simulink model "Full_avg_converter"  (R2023b)
settings: Solver=VariableStepAuto  StartTime=0.0  StopTime=sim_time  RelTol=1e-3
undefined symbols (not defined in the file or in its folder): Bat, boost, ccm_mpp_reg_param, ccm_reg_param, dcm_mpp_reg_param, dcm_reg_param, m0_ccm, mppt_my3, pv_data, pv_eq, Ramp, sim_op, Tmfc, Uoc_max, Uref
libraries: spsBistableLib x3, slpidlib x3, simulink x1, spspowerguiLib x1
settings Model: Creator=teo  LastModifiedBy=teo

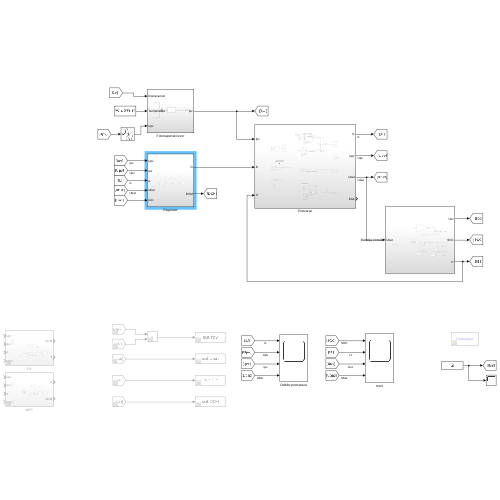
[thumbnail: Simulink's stored preview of the top-level diagram]
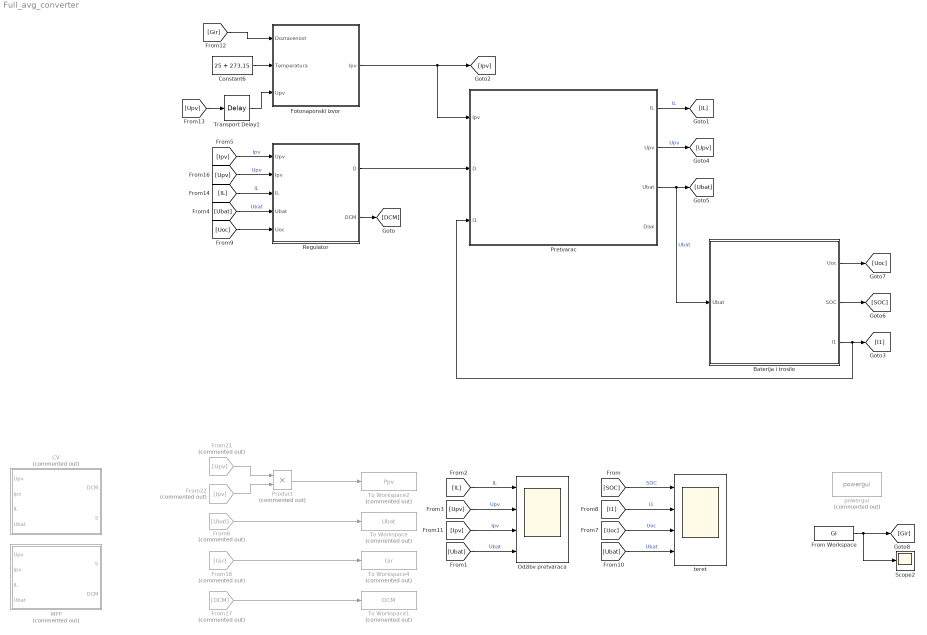
== system Full_avg_converter ==
  Baterija i trosilo : Subsystem
  CV : Subsystem  Commented=on
  Constant6 : Constant  Value=25 + 273.15
  Fotonaponski izvor : Subsystem
  From Workspace : FromWorkspace  VariableName=GI
  From17 : From  Commented=on  GotoTag=DCM
  From18 : From  Commented=on  GotoTag=Gir
  From21 : From  Commented=on  GotoTag=Upv
  From22 : From  Commented=on  GotoTag=Ipv
  From6 : From  Commented=on  GotoTag=Ubat
  MPP : Subsystem  Commented=on
  Odzibv pretvaraca : Scope  NumInputPorts=4
  Pretvarac : Subsystem
  Product : Product  Commented=on
  Regulator : Subsystem
  Scope2 : Scope
  To Workspace : ToWorkspace  Commented=on  VariableName=Ubat  SaveFormat=Timeseries  SampleTime=-1
  To Workspace1 : ToWorkspace  Commented=on  VariableName=DCM  SaveFormat=Timeseries  SampleTime=-1
  To Workspace2 : ToWorkspace  Commented=on  VariableName=Ppv  SaveFormat=Timeseries  SampleTime=-1
  To Workspace4 : ToWorkspace  Commented=on  VariableName=Gir  SaveFormat=Timeseries  SampleTime=-1
  Transport Delay1 : TransportDelay  DelayTime=0.0001  BufferSize=4024
  powergui : spspowerguiLib/powergui  Priority=1  Commented=on  SimulationMode=Continuous  SampleTime=50e-6  frequency=60  Iterations=50  frequencyindice=0  Pbase=100e6  ErrMax=1e-4  UnitsV=kV  UnitsW=MW  buscounter=0  FunctionMessages=off  echomessages=off  EnableUseOfTLC=off  CurrentSourceSwitches=off  DisableSnubberDevices=off  DisableRonSwitches=off  DisableVfSwitches=off  DisplayEquations=off  AutomaticDiscreteSolvers=off  SolverType=Tustin/Backward Euler (TBE)  Interpol=off  ExternalGateDelay=off  methode=off  Ts=100  x0status=blocks  SPID=on  SwTol=0  HookPort=off  NonlinearTolerance=1e-4  nMaxIteration=100  ContinueOnMaxIteration=off  RestoreLinks=warning  ResistiveCurrentMeasurement=off  Frange=[0:2:500]  Ylog=off  Xlog=on  ShowGrid=off  save=off  variable=ZData  structure=0  ZoomFFT=off  StartTime=0.0  cycles=1  DisplayStyle=1  fundamental=60  FreqAxis=off  MaxFrequency=1000  frequencyindicesteady=1  RmsSteady=1  display=off
  teret : Scope  NumInputPorts=4
  wires:
  Product/1 -> To Workspace2/1
  [I1] -> teret/2  "I1"
  Transport Delay1/1 -> Fotonaponski izvor/3(Upv)
  [Ubat] -> Odzibv pretvaraca/4  "Ubat"
  Constant6/1 -> Fotonaponski izvor/2(Temperatura)
  [Upv] -> Odzibv pretvaraca/2  "Upv"
  From Workspace/1 -> Scope2/1, [Gir]
  [Upv] -> Transport Delay1/1
  [Ipv] -> Odzibv pretvaraca/3  "Ipv"
  [Ubat] -> teret/4  "Ubat"
  From18/1 -> To Workspace4/1
  [IL] -> Odzibv pretvaraca/1  "IL"
  From6/1 -> To Workspace/1
  From17/1 -> To Workspace1/1
  From21/1 -> Product/1
  From22/1 -> Product/2
  Regulator/1(D) -> Pretvarac/2(D)
  Regulator/2(DCM) -> [DCM]
  [IL] -> Regulator/3(IL)  "IL"
  [Ubat] -> Regulator/4(Ubat)  "Ubat"
  [Upv] -> Regulator/2(Ipv)  "Upv"
  [Ipv] -> Regulator/1(Upv)  "Ipv"
  Pretvarac/1(IL) -> [IL]  "IL"
  Pretvarac/2(Upv) -> [Upv]  "Upv"
  Pretvarac/3(Ubat) -> Baterija i trosilo/1(Ubat), [Ubat]  "Ubat"
  Baterija i trosilo/3(I1) -> [I1], Pretvarac/3(I1)
  Baterija i trosilo/2(SOC) -> [SOC]
  Fotonaponski izvor/1(Ipv) -> [Ipv], Pretvarac/1(Ipv)
  Baterija i trosilo/1(Uoc) -> [Uoc]
  [Uoc] -> Regulator/5(Uoc)
  [SOC] -> teret/1  "SOC"
  [Uoc] -> teret/3  "Uoc"
  [Gir] -> Fotonaponski izvor/1(Dozracenost)

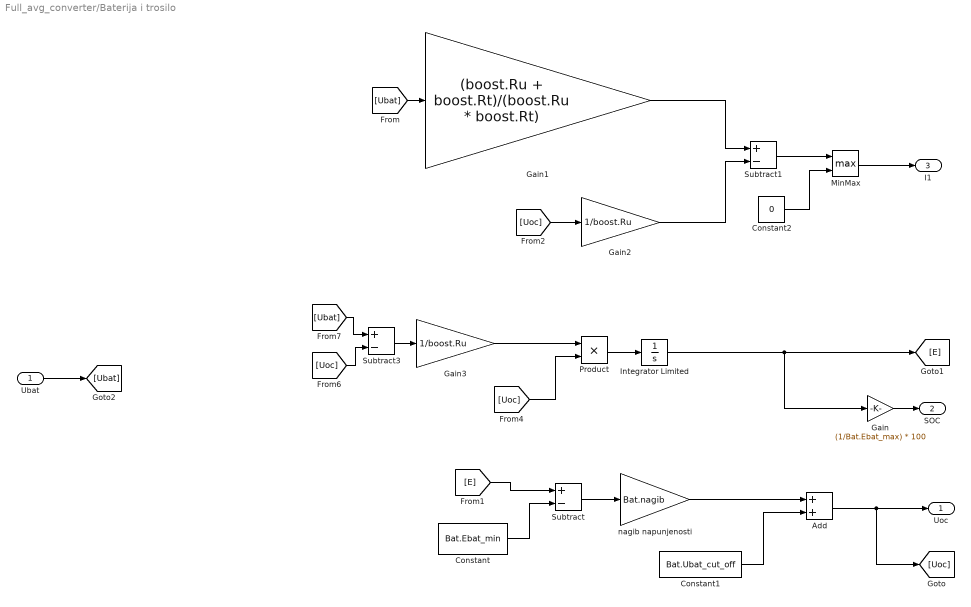
== system Full_avg_converter/Baterija i trosilo ==
  Ubat : Inport
  Add : Sum
  Constant : Constant  Value=Bat.Ebat_min
  Constant1 : Constant  Value=Bat.Ubat_cut_off
  Constant2 : Constant  Value=0
  Gain : Gain  Gain=(1/Bat.Ebat_max) * 100
  Gain1 : Gain  Gain=(boost.Ru + boost.Rt)/(boost.Ru * boost.Rt)
  Gain2 : Gain  Gain=1/boost.Ru
  Gain3 : Gain  Gain=1/boost.Ru
  Integrator Limited : Integrator  InitialCondition=sim_op.E0  LimitOutput=on  UpperSaturationLimit=Bat.Ebat_max  LowerSaturationLimit=Bat.Ebat_min
  MinMax : MinMax  Function=max  Inputs=2
  Product : Product
  Subtract : Sum  Inputs=+-
  Subtract1 : Sum  Inputs=+-
  Subtract3 : Sum  Inputs=+-
  nagib napunjenosti : Gain  Gain=Bat.nagib
  Uoc : Outport
  SOC : Outport  Port=2
  I1 : Outport  Port=3
  wires:
  Subtract/1 -> nagib napunjenosti/1
  Constant/1 -> Subtract/2
  nagib napunjenosti/1 -> Add/1
  Constant1/1 -> Add/2
  Integrator Limited/1 -> Gain/1, [E]
  [Uoc] -> Product/2
  Product/1 -> Integrator Limited/1
  [E] -> Subtract/1
  Gain/1 -> SOC/1
  Add/1 -> Uoc/1, [Uoc]
  Ubat/1 -> [Ubat]
  [Ubat] -> Gain1/1
  Gain1/1 -> Subtract1/1
  [Uoc] -> Gain2/1
  Gain2/1 -> Subtract1/2
  MinMax/1 -> I1/1
  Subtract1/1 -> MinMax/1
  Constant2/1 -> MinMax/2
  Subtract3/1 -> Gain3/1
  Gain3/1 -> Product/1
  [Ubat] -> Subtract3/1
  [Uoc] -> Subtract3/2

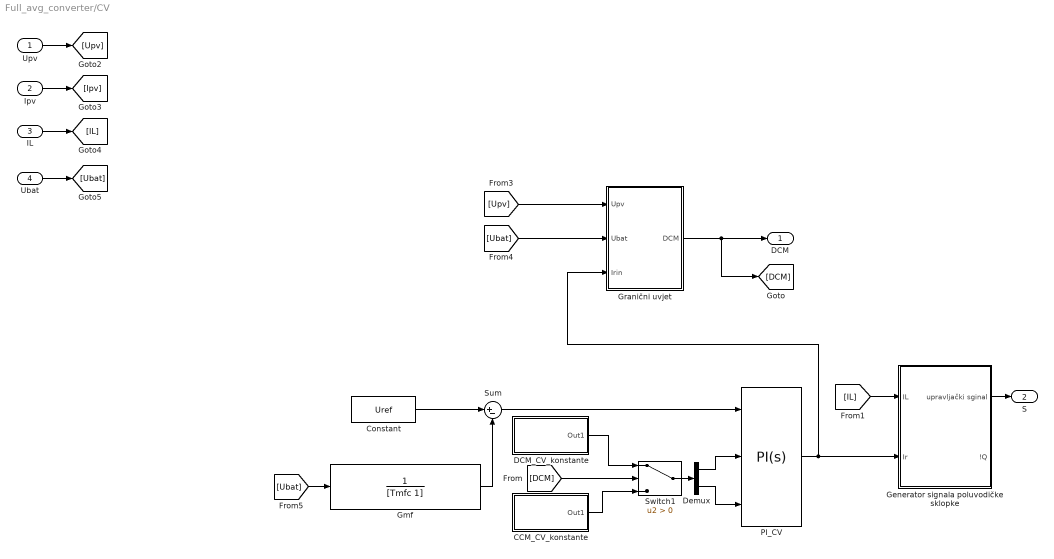
== system Full_avg_converter/CV ==
  Upv : Inport
  Ipv : Inport  Port=2
  IL : Inport  Port=3
  Ubat : Inport  Port=4
  CCM_CV_konstante : Subsystem
  Constant : Constant  Value=Uref
  DCM_CV_konstante : Subsystem
  Demux : Demux  Outputs=2
  Generator signala poluvodičke sklopke : Subsystem
  Gmf : TransferFcn  Numerator=1  Denominator=[Tmfc 1]
  Granični uvjet : Subsystem
  PI_CV : slpidlib/PID Controller  Controller=PI  Form=Parallel  TimeDomain=Continuous-time  UseExternalTs=off  SampleTime=-1  IntegratorMethod=Forward Euler  FilterMethod=Forward Euler  ControllerParametersSource=external  P=ccm_mpp_reg_param.KR  I=ccm_mpp_reg_param.KR/ccm_mpp_reg_param.Ti  UseKiTs=off  D=0  N=100  UseFilter=on  TunerSelectOption=Transfer Function Based (PID Tuner App)  InitialConditionSource=internal  InitialConditionForIntegrator=0  InitialConditionForFilter=0  DifferentiatorICPrevScaledInput=0  ExternalReset=none  TrackingMode=off  Kt=1  LimitOutput=on  SatLimitsSource=internal  UpperSaturationLimit=2  LowerSaturationLimit=-2  LinearizeAsGain=off  AntiWindupMode=clamping  Kb=1  LimitIntegrator=off  UpperIntegratorSaturationLimit=inf  LowerIntegratorSaturationLimit=-inf  POutMin=[]  POutMax=[]  IOutMin=[]  IOutMax=[]  DOutMin=[]  DOutMax=[]  NOutMin=[]  NOutMax=[]  SumOutMin=[]  SumOutMax=[]  SaturationOutMin=[]  SaturationOutMax=[]  PParamMin=[]  PParamMax=[]  IParamMin=[]  IParamMax=[]  DParamMin=[]  DParamMax=[]  NParamMin=[]  NParamMax=[]  KbParamMin=[]  KbParamMax=[]  KtParamMin=[]  KtParamMax=[]  KbOutMin=[]  KbOutMax=[]  KtOutMin=[]  KtOutMax=[]  IntegratorOutMin=[]  IntegratorOutMax=[]  FilterOutMin=[]  FilterOutMax=[]  SumI1OutMin=[]  SumI1OutMax=[]  SumI2OutMin=[]  SumI2OutMax=[]  SumI3OutMin=[]  SumI3OutMax=[]  SumI4OutMin=[]  SumI4OutMax=[]  SumDOutMin=[]  SumDOutMax=[]  DifferentiatorOutMin=[]  DifferentiatorOutMax=[]  FilterDiffOutCoefMin=[]  FilterDiffOutCoefMax=[]  ReciprocalOutMin=[]  ReciprocalOutMax=[]  SumDenOutMin=[]  SumDenOutMax=[]  SumNumOutMin=[]  SumNumOutMax=[]  DivideOutMin=[]  DivideOutMax=[]  UdiffTsProdOutMin=[]  UdiffTsProdOutMax=[]  NTsProdOutMin=[]  NTsProdOutMax=[]  UintegralTsProdOutMin=[]  UintegralTsProdOutMax=[]  UngainTsProdOutMin=[]  UngainTsProdOutMax=[]  ClampingZeroOutDataTypeStr=Inherit: Inherit via back propagation  ClampingZeroOutMin=[]  ClampingZeroOutMax=[]  FilterDenConstantOutDataTypeStr=Inherit: Inherit via back propagation  FilterDenConstantOutMin=[]  FilterDenConstantOutMax=[]  PCopyOutDataTypeStr=Inherit: Inherit via back propagation  PCopyOutMin=[]  PCopyOutMax=[]  NCopyOutDataTypeStr=Inherit: Inherit via back propagation  NCopyOutMin=[]  NCopyOutMax=[]  IntegratorContinuousStateAttributes=''  IntegratorStateMustResolveToSignalObject=off  IntegratorRTWStateStorageClass=Auto  FilterContinuousStateAttributes=''  FilterStateMustResolveToSignalObject=off  FilterRTWStateStorageClass=Auto  ParallelPVariant=ExternalParameters  IdealPVariant=Disabled  IVariant=ExternalParameters  DVariant=Disabled  IntegratorVariant=Continuous  SatVariant=Enabled  AWVariant=ContClampingParallel  PCopyVariant=Disabled  TRVariant=Disabled  FdbkBlocksVariant=Forward  IdealPFdbkVariant=Disabled  SatFdbkVariant=Disabled  DerivativeFilterVariant=Disabled  NVariant=Disabled  NCopyVariant=Disabled_SignalSpec  FilterICVariant=Disabled  IntegratorICVariant=InternalICs  ExternalResetVariant=Disabled  TRSumVariant=Passthrough  SumFdbkVariant=Disabled  SumVariant=Sum_PI  TsampFilterVariant=InternalTs  TsampNgainVariant=Passthrough  TsampIntegralVariant=Disabled_SignalSpec  ExternalSaturationOutDataTypeStr=Inherit: Same as second input
  Sum : Sum  Inputs=|+-
  Switch1 : Switch  Criteria=u2 > Threshold  SaturateOnIntegerOverflow=off  InputSameDT=off
  DCM : Outport
  S : Outport  Port=2
  wires:
  Switch1/1 -> Demux/1
  Demux/1 -> PI_CV/2
  Demux/2 -> PI_CV/3
  [DCM] -> Switch1/2
  DCM_CV_konstante/1(Out1) -> Switch1/1
  CCM_CV_konstante/1(Out1) -> Switch1/3
  Generator signala poluvodičke sklopke/1(upravljački sginal) -> S/1
  Upv/1 -> [Upv]
  Ipv/1 -> [Ipv]
  Ubat/1 -> [Ubat]
  IL/1 -> [IL]
  Granični uvjet/1(DCM) -> [DCM], DCM/1
  [Upv] -> Granični uvjet/1(Upv)
  [Ubat] -> Granični uvjet/2(Ubat)
  PI_CV/1 -> Generator signala poluvodičke sklopke/2(Ir), Granični uvjet/3(Irin)
  [IL] -> Generator signala poluvodičke sklopke/1(IL)
  [Ubat] -> Gmf/1
  Constant/1 -> Sum/1
  Gmf/1 -> Sum/2
  Sum/1 -> PI_CV/1

== system Full_avg_converter/Fotonaponski izvor ==
  Dozracenost : Inport
  Temperatura : Inport  Port=2
  Upv : Inport  Port=3
  Fotonaponsko polje : MATLABFcn  MATLABFcn=pv_eq(u(1), u(2), [], u(3), pv_data, 1, 1)  OutputDimensions=1
  Mux : Mux  Inputs=3
  Ipv : Outport
  wires:
  Fotonaponsko polje/1 -> Ipv/1  "Ipv"
  Mux/1 -> Fotonaponsko polje/1
  Dozracenost/1 -> Mux/1
  Temperatura/1 -> Mux/2
  Upv/1 -> Mux/3

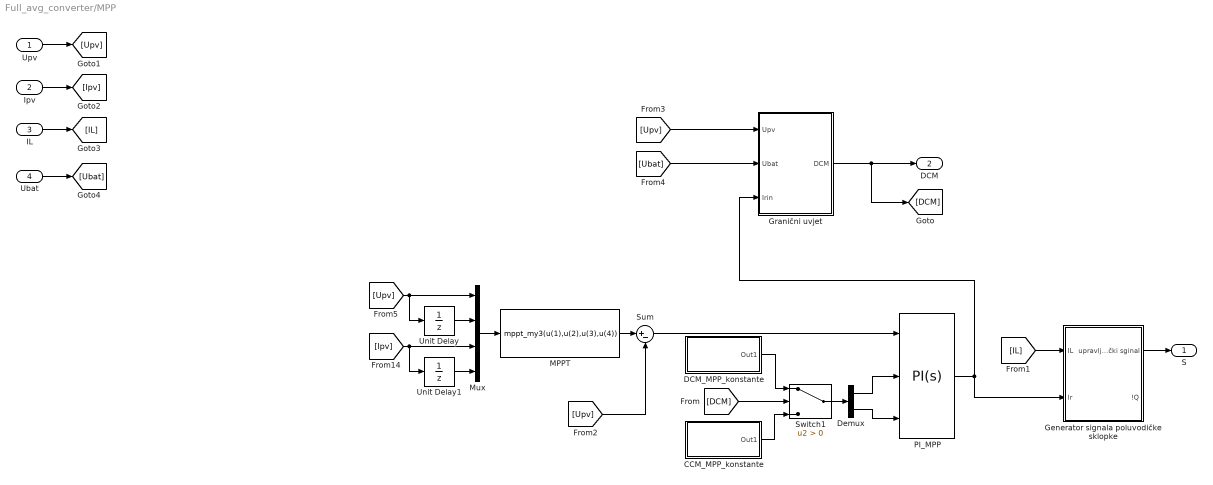
== system Full_avg_converter/MPP ==
  Upv : Inport
  Ipv : Inport  Port=2
  IL : Inport  Port=3
  Ubat : Inport  Port=4
  CCM_MPP_konstante : Subsystem
  DCM_MPP_konstante : Subsystem
  Demux : Demux  Outputs=2
  Generator signala poluvodičke sklopke : Subsystem
  Granični uvjet : Subsystem
  MPPT : MATLABFcn  MATLABFcn=mppt_my3(u(1),u(2),u(3),u(4))
  Mux : Mux
  PI_MPP : slpidlib/PID Controller  Controller=PI  Form=Parallel  TimeDomain=Continuous-time  UseExternalTs=off  SampleTime=-1  IntegratorMethod=Forward Euler  FilterMethod=Forward Euler  ControllerParametersSource=external  P=ccm_mpp_reg_param.KR  I=ccm_mpp_reg_param.KR/ccm_mpp_reg_param.Ti  UseKiTs=off  D=0  N=100  UseFilter=on  TunerSelectOption=Transfer Function Based (PID Tuner App)  InitialConditionSource=internal  InitialConditionForIntegrator=0  InitialConditionForFilter=0  DifferentiatorICPrevScaledInput=0  ExternalReset=none  TrackingMode=off  Kt=1  LimitOutput=on  SatLimitsSource=internal  UpperSaturationLimit=2  LowerSaturationLimit=-2  LinearizeAsGain=off  AntiWindupMode=clamping  Kb=1  LimitIntegrator=off  UpperIntegratorSaturationLimit=inf  LowerIntegratorSaturationLimit=-inf  POutMin=[]  POutMax=[]  IOutMin=[]  IOutMax=[]  DOutMin=[]  DOutMax=[]  NOutMin=[]  NOutMax=[]  SumOutMin=[]  SumOutMax=[]  SaturationOutMin=[]  SaturationOutMax=[]  PParamMin=[]  PParamMax=[]  IParamMin=[]  IParamMax=[]  DParamMin=[]  DParamMax=[]  NParamMin=[]  NParamMax=[]  KbParamMin=[]  KbParamMax=[]  KtParamMin=[]  KtParamMax=[]  KbOutMin=[]  KbOutMax=[]  KtOutMin=[]  KtOutMax=[]  IntegratorOutMin=[]  IntegratorOutMax=[]  FilterOutMin=[]  FilterOutMax=[]  SumI1OutMin=[]  SumI1OutMax=[]  SumI2OutMin=[]  SumI2OutMax=[]  SumI3OutMin=[]  SumI3OutMax=[]  SumI4OutMin=[]  SumI4OutMax=[]  SumDOutMin=[]  SumDOutMax=[]  DifferentiatorOutMin=[]  DifferentiatorOutMax=[]  FilterDiffOutCoefMin=[]  FilterDiffOutCoefMax=[]  ReciprocalOutMin=[]  ReciprocalOutMax=[]  SumDenOutMin=[]  SumDenOutMax=[]  SumNumOutMin=[]  SumNumOutMax=[]  DivideOutMin=[]  DivideOutMax=[]  UdiffTsProdOutMin=[]  UdiffTsProdOutMax=[]  NTsProdOutMin=[]  NTsProdOutMax=[]  UintegralTsProdOutMin=[]  UintegralTsProdOutMax=[]  UngainTsProdOutMin=[]  UngainTsProdOutMax=[]  ClampingZeroOutDataTypeStr=Inherit: Inherit via back propagation  ClampingZeroOutMin=[]  ClampingZeroOutMax=[]  FilterDenConstantOutDataTypeStr=Inherit: Inherit via back propagation  FilterDenConstantOutMin=[]  FilterDenConstantOutMax=[]  PCopyOutDataTypeStr=Inherit: Inherit via back propagation  PCopyOutMin=[]  PCopyOutMax=[]  NCopyOutDataTypeStr=Inherit: Inherit via back propagation  NCopyOutMin=[]  NCopyOutMax=[]  IntegratorContinuousStateAttributes=''  IntegratorStateMustResolveToSignalObject=off  IntegratorRTWStateStorageClass=Auto  FilterContinuousStateAttributes=''  FilterStateMustResolveToSignalObject=off  FilterRTWStateStorageClass=Auto  ParallelPVariant=ExternalParameters  IdealPVariant=Disabled  IVariant=ExternalParameters  DVariant=Disabled  IntegratorVariant=Continuous  SatVariant=Enabled  AWVariant=ContClampingParallel  PCopyVariant=Disabled  TRVariant=Disabled  FdbkBlocksVariant=Forward  IdealPFdbkVariant=Disabled  SatFdbkVariant=Disabled  DerivativeFilterVariant=Disabled  NVariant=Disabled  NCopyVariant=Disabled_SignalSpec  FilterICVariant=Disabled  IntegratorICVariant=InternalICs  ExternalResetVariant=Disabled  TRSumVariant=Passthrough  SumFdbkVariant=Disabled  SumVariant=Sum_PI  TsampFilterVariant=InternalTs  TsampNgainVariant=Passthrough  TsampIntegralVariant=Disabled_SignalSpec  ExternalSaturationOutDataTypeStr=Inherit: Same as second input
  Sum : Sum  Inputs=|+-
  Switch1 : Switch  Criteria=u2 > Threshold  SaturateOnIntegerOverflow=off  InputSameDT=off
  Unit Delay : UnitDelay  SampleTime=-1  HasFrameUpgradeWarning=on
  Unit Delay1 : UnitDelay  SampleTime=-1  HasFrameUpgradeWarning=on
  S : Outport
  DCM : Outport  Port=2
  wires:
  Switch1/1 -> Demux/1
  Demux/1 -> PI_MPP/2
  Demux/2 -> PI_MPP/3
  [DCM] -> Switch1/2
  DCM_MPP_konstante/1(Out1) -> Switch1/1
  CCM_MPP_konstante/1(Out1) -> Switch1/3
  PI_MPP/1 -> Granični uvjet/3(Irin), Generator signala poluvodičke sklopke/2(Ir)
  Generator signala poluvodičke sklopke/1(upravljački sginal) -> S/1
  Mux/1 -> MPPT/1
  Granični uvjet/1(DCM) -> [DCM], DCM/1
  MPPT/1 -> Sum/1
  [Upv] -> Sum/2
  Unit Delay/1 -> Mux/2
  Unit Delay1/1 -> Mux/4
  Sum/1 -> PI_MPP/1
  Upv/1 -> [Upv]
  Ipv/1 -> [Ipv]
  IL/1 -> [IL]
  Ubat/1 -> [Ubat]
  [IL] -> Generator signala poluvodičke sklopke/1(IL)
  [Upv] -> Granični uvjet/1(Upv)
  [Ubat] -> Granični uvjet/2(Ubat)
  [Upv] -> Unit Delay/1, Mux/1
  [Ipv] -> Unit Delay1/1, Mux/3

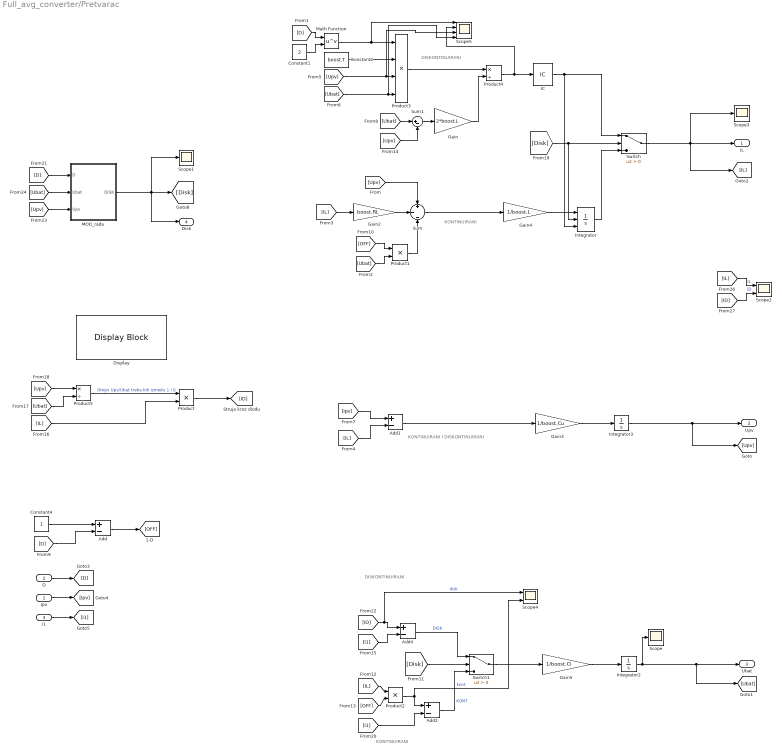
== system Full_avg_converter/Pretvarac ==
  note: DISKONTINUIRANI
  note: KONTINUIRANI
  note: KONTINUIRANI I DISKONTINUIRANI
  note: KONTINUIRANI
  note: DISKONTINUIRANI
  Ipv : Inport
  D : Inport  Port=2
  I1 : Inport  Port=3
  Add{,1..2,4} (4 alike) : Sum  Inputs=+-
  Constant1 : Constant  Value=2
  Constant2 : Constant  Value=boost.T
  Constant4 : Constant
  Display : DisplayBlock  LabelPosition=Bottom  Transparency=1
  Gain : Gain  Gain=2*boost.L
  Gain2 : Gain  Gain=boost.RL
  Gain3 : Gain  Gain=1/boost.Cu
  Gain4 : Gain  Gain=1/boost.L
  Gain5 : Gain  Gain=1/boost.Ci
  IC : InitialCondition  Value=0.1
  Integrator : Integrator  ExternalReset=falling  InitialConditionSource=external  LimitOutput=on  UpperSaturationLimit=150  LowerSaturationLimit=0
  Integrator2 : Integrator  InitialCondition=0.2  UpperSaturationLimit=Uoc_max + 10  LowerSaturationLimit=0
  Integrator3 : Integrator  InitialCondition=0.1  LimitOutput=on  UpperSaturationLimit=pv_data.Uoc  LowerSaturationLimit=0
  MOD_rada : Subsystem
  Math Function : Math  Operator=pow
  Product : Product
  Product1 : Product
  Product2 : Product
  Product3 : Product  Inputs=4
  Product4 : Product  Inputs=*/
  Product5 : Product  Inputs=*/
  Scope : Scope
  Scope1 : Scope
  Scope2 : Scope  NumInputPorts=2
  Scope3 : Scope
  Scope4 : Scope  NumInputPorts=2
  Scope5 : Scope  NumInputPorts=4
  Sum : Sum  Inputs=+|-|-
  Sum1 : Sum  Inputs=|+-
  Switch : Switch  Criteria=u2 > Threshold  SaturateOnIntegerOverflow=off  InputSameDT=off
  Switch1 : Switch  Criteria=u2 > Threshold  SaturateOnIntegerOverflow=off  InputSameDT=off
  IL : Outport
  Upv : Outport  Port=2
  Ubat : Outport  Port=3
  Disk : Outport  Port=4
  wires:
  I1/1 -> [I1]
  [Ipv] -> Add1/1
  D/1 -> [D]
  Ipv/1 -> [Ipv]
  [Upv] -> Sum/1
  [D] -> Add/2
  Constant4/1 -> Add/1
  Product1/1 -> Sum/3
  [OFF] -> Product1/1
  [Ubat] -> Product1/2
  [IL] -> Add1/2
  Sum/1 -> Gain4/1
  Add1/1 -> Gain3/1
  [D] -> Math Function/1
  Constant1/1 -> Math Function/2
  Math Function/1 -> Scope5/1, Product3/1
  Constant2/1 -> Product3/2
  [Upv] -> Scope5/3, Product3/3
  [Ubat] -> Scope5/4, Product3/4
  Product3/1 -> Product4/1
  [Ubat] -> Sum1/1
  [Upv] -> Sum1/2
  Sum1/1 -> Gain/1
  Gain3/1 -> Integrator3/1
  Gain/1 -> Product4/2
  Switch/1 -> Scope3/1, IL/1, [IL]
  Add/1 -> [OFF]
  Gain2/1 -> Sum/2
  [IL] -> Gain2/1
  Gain5/1 -> Integrator2/1
  [D] -> MOD_rada/1(D)
  [Upv] -> MOD_rada/3(Upv)
  [Ubat] -> MOD_rada/2(Ubat)
  Integrator3/1 -> [Upv], Upv/1
  Gain4/1 -> Integrator/1
  Integrator/1 -> Switch/3
  [Disk] -> Integrator/2, Switch/2
  [Upv] -> Product5/1
  [Ubat] -> Product5/2
  [IL] -> Product/2
  Product/1 -> [ID]
  Product5/1 -> Product/1  "Omjer Upv/Ubat treba biti izmedu 1 i 0"
  [ID] -> Scope4/1, Add4/1  "disk"
  [I1] -> Add4/2
  [IL] -> Scope2/1  "IL"
  [ID] -> Scope2/2  "ID"
  IC/1 -> Integrator/3, Switch/1
  Switch1/1 -> Gain5/1
  Add4/1 -> Switch1/1  "DISK"
  [Disk] -> Switch1/2
  [IL] -> Product2/1
  [OFF] -> Product2/2
  Product2/1 -> Add2/1, Scope4/2  "kont"
  [I1] -> Add2/2
  Add2/1 -> Switch1/3  "KONT"
  MOD_rada/1(DISK) -> Disk/1, Scope1/1, [Disk]
  Integrator2/1 -> [Ubat], Ubat/1, Scope/1
  Product4/1 -> Scope5/2, IC/1

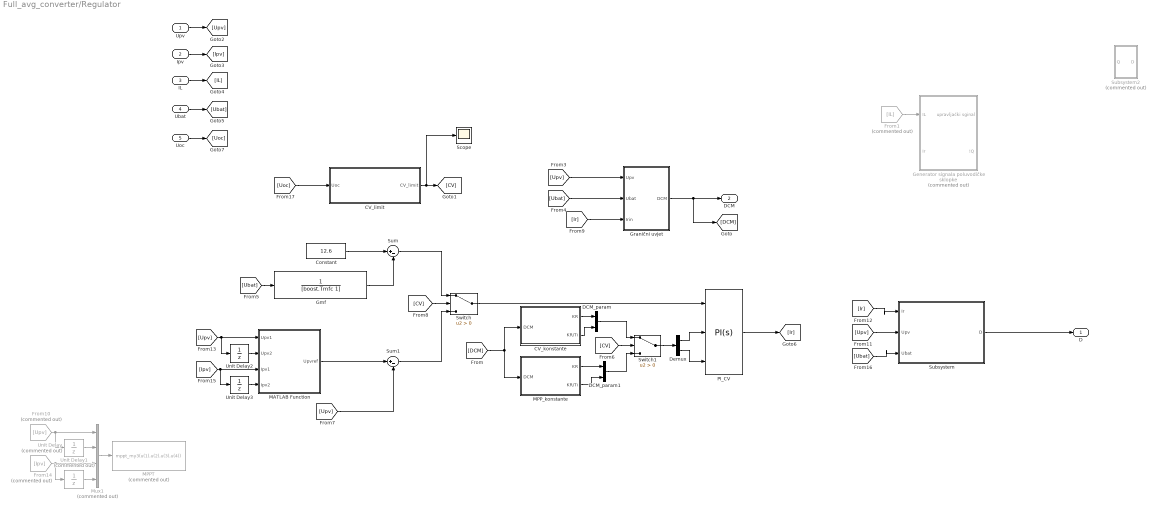
== system Full_avg_converter/Regulator ==
  Upv : Inport
  Ipv : Inport  Port=2
  IL : Inport  Port=3
  Ubat : Inport  Port=4
  Uoc : Inport  Port=5
  CV_konstante : Subsystem
  CV_limit : Subsystem
  Constant : Constant  Value=12.6
  DCM_param : Mux  Inputs=2
  DCM_param1 : Mux  Inputs=2
  Demux : Demux  Outputs=2
  From1 : From  Commented=on  GotoTag=IL
  From10 : From  Commented=on  GotoTag=Upv
  From14 : From  Commented=on  GotoTag=Ipv
  Generator signala poluvodičke sklopke : Subsystem  Commented=on
  Gmf : TransferFcn  Numerator=1  Denominator=[boost.Tmfc 1]
  Granični uvjet : Subsystem
  MATLAB Function : MATLAB Function  TreatAsAtomicUnit=on
  MPPT : MATLABFcn  Commented=on  MATLABFcn=mppt_my3(u(1),u(2),u(3),u(4))
  MPP_konstante : Subsystem
  Mux1 : Mux  Commented=on
  PI_CV : slpidlib/PID Controller  Controller=PI  Form=Parallel  TimeDomain=Continuous-time  UseExternalTs=off  SampleTime=-1  IntegratorMethod=Forward Euler  FilterMethod=Forward Euler  ControllerParametersSource=external  P=ccm_mpp_reg_param.KR  I=ccm_mpp_reg_param.KR/ccm_mpp_reg_param.Ti  UseKiTs=off  D=0  N=100  UseFilter=on  TunerSelectOption=Transfer Function Based (PID Tuner App)  InitialConditionSource=internal  InitialConditionForIntegrator=0  InitialConditionForFilter=0  DifferentiatorICPrevScaledInput=0  ExternalReset=none  TrackingMode=off  Kt=1  LimitOutput=on  SatLimitsSource=internal  UpperSaturationLimit=2  LowerSaturationLimit=-2  LinearizeAsGain=off  AntiWindupMode=clamping  Kb=1  LimitIntegrator=off  UpperIntegratorSaturationLimit=inf  LowerIntegratorSaturationLimit=-inf  POutMin=[]  POutMax=[]  IOutMin=[]  IOutMax=[]  DOutMin=[]  DOutMax=[]  NOutMin=[]  NOutMax=[]  SumOutMin=[]  SumOutMax=[]  SaturationOutMin=[]  SaturationOutMax=[]  PParamMin=[]  PParamMax=[]  IParamMin=[]  IParamMax=[]  DParamMin=[]  DParamMax=[]  NParamMin=[]  NParamMax=[]  KbParamMin=[]  KbParamMax=[]  KtParamMin=[]  KtParamMax=[]  KbOutMin=[]  KbOutMax=[]  KtOutMin=[]  KtOutMax=[]  IntegratorOutMin=[]  IntegratorOutMax=[]  FilterOutMin=[]  FilterOutMax=[]  SumI1OutMin=[]  SumI1OutMax=[]  SumI2OutMin=[]  SumI2OutMax=[]  SumI3OutMin=[]  SumI3OutMax=[]  SumI4OutMin=[]  SumI4OutMax=[]  SumDOutMin=[]  SumDOutMax=[]  DifferentiatorOutMin=[]  DifferentiatorOutMax=[]  FilterDiffOutCoefMin=[]  FilterDiffOutCoefMax=[]  ReciprocalOutMin=[]  ReciprocalOutMax=[]  SumDenOutMin=[]  SumDenOutMax=[]  SumNumOutMin=[]  SumNumOutMax=[]  DivideOutMin=[]  DivideOutMax=[]  UdiffTsProdOutMin=[]  UdiffTsProdOutMax=[]  NTsProdOutMin=[]  NTsProdOutMax=[]  UintegralTsProdOutMin=[]  UintegralTsProdOutMax=[]  UngainTsProdOutMin=[]  UngainTsProdOutMax=[]  ClampingZeroOutDataTypeStr=Inherit: Inherit via back propagation  ClampingZeroOutMin=[]  ClampingZeroOutMax=[]  FilterDenConstantOutDataTypeStr=Inherit: Inherit via back propagation  FilterDenConstantOutMin=[]  FilterDenConstantOutMax=[]  PCopyOutDataTypeStr=Inherit: Inherit via back propagation  PCopyOutMin=[]  PCopyOutMax=[]  NCopyOutDataTypeStr=Inherit: Inherit via back propagation  NCopyOutMin=[]  NCopyOutMax=[]  IntegratorContinuousStateAttributes=''  IntegratorStateMustResolveToSignalObject=off  IntegratorRTWStateStorageClass=Auto  FilterContinuousStateAttributes=''  FilterStateMustResolveToSignalObject=off  FilterRTWStateStorageClass=Auto  ParallelPVariant=ExternalParameters  IdealPVariant=Disabled  IVariant=ExternalParameters  DVariant=Disabled  IntegratorVariant=Continuous  SatVariant=Enabled  AWVariant=ContClampingParallel  PCopyVariant=Disabled  TRVariant=Disabled  FdbkBlocksVariant=Forward  IdealPFdbkVariant=Disabled  SatFdbkVariant=Disabled  DerivativeFilterVariant=Disabled  NVariant=Disabled  NCopyVariant=Disabled_SignalSpec  FilterICVariant=Disabled  IntegratorICVariant=InternalICs  ExternalResetVariant=Disabled  TRSumVariant=Passthrough  SumFdbkVariant=Disabled  SumVariant=Sum_PI  TsampFilterVariant=InternalTs  TsampNgainVariant=Passthrough  TsampIntegralVariant=Disabled_SignalSpec  ExternalSaturationOutDataTypeStr=Inherit: Same as second input
  Scope : Scope
  Subsystem : Subsystem
  Subsystem2 : Subsystem  Commented=on
  Sum : Sum  Inputs=|+-
  Sum1 : Sum  Inputs=|+-
  Switch : Switch  Criteria=u2 > Threshold  SaturateOnIntegerOverflow=off  InputSameDT=off
  Switch1 : Switch  Criteria=u2 > Threshold  SaturateOnIntegerOverflow=off  InputSameDT=off
  Unit Delay : UnitDelay  Commented=on  SampleTime=-1  HasFrameUpgradeWarning=on
  Unit Delay1 : UnitDelay  Commented=on  SampleTime=-1  HasFrameUpgradeWarning=on
  Unit Delay2 : UnitDelay  SampleTime=-1  HasFrameUpgradeWarning=on
  Unit Delay3 : UnitDelay  SampleTime=-1  HasFrameUpgradeWarning=on
  D : Outport
  DCM : Outport  Port=2
  wires:
  Switch1/1 -> Demux/1
  Demux/1 -> PI_CV/2
  Demux/2 -> PI_CV/3
  Upv/1 -> [Upv]
  Ipv/1 -> [Ipv]
  Ubat/1 -> [Ubat]
  IL/1 -> [IL]
  Granični uvjet/1(DCM) -> [DCM], DCM/1
  [Ubat] -> Granični uvjet/2(Ubat)
  From1/1 -> Generator signala poluvodičke sklopke/1(IL)
  [Ubat] -> Gmf/1
  Constant/1 -> Sum/1
  Gmf/1 -> Sum/2
  Unit Delay1/1 -> Mux1/4
  Unit Delay/1 -> Mux1/2
  [Upv] -> Sum1/2
  Mux1/1 -> MPPT/1
  From10/1 -> Mux1/1, Unit Delay/1
  From14/1 -> Mux1/3, Unit Delay1/1
  [DCM] -> MPP_konstante/1(DCM), CV_konstante/1(DCM)
  [Uoc] -> CV_limit/1(Uoc)
  [Upv] -> Granični uvjet/1(Upv)
  CV_limit/1(CV_limit) -> Scope/1, [CV]
  [CV] -> Switch1/2
  [CV] -> Switch/2
  Sum/1 -> Switch/1
  [Ir] -> Granični uvjet/3(Irin)
  CV_konstante/1(KR) -> DCM_param/1
  CV_konstante/2(KR/Ti) -> DCM_param/2
  DCM_param/1 -> Switch1/1
  MPP_konstante/1(KR) -> DCM_param1/1
  MPP_konstante/2(KR/Ti) -> DCM_param1/2
  DCM_param1/1 -> Switch1/3
  [Ir] -> Subsystem/1(Ir)
  [Upv] -> Subsystem/2(Upv)
  [Ubat] -> Subsystem/3(Ubat)
  PI_CV/1 -> [Ir]
  Sum1/1 -> Switch/3
  Switch/1 -> PI_CV/1
  MATLAB Function/1(Upvref) -> Sum1/1
  Unit Delay3/1 -> MATLAB Function/4(Ipv2)
  [Ipv] -> MATLAB Function/3(Ipv1), Unit Delay3/1
  [Upv] -> MATLAB Function/1(Upv1), Unit Delay2/1
  Unit Delay2/1 -> MATLAB Function/2(Upv2)
  Uoc/1 -> [Uoc]
  Subsystem/1(D) -> D/1

== system Full_avg_converter/CV/CCM_CV_konstante ==
  Constant : Constant  Value=ccm_reg_param.KR
  Constant1 : Constant  Value=ccm_reg_param.KR/ccm_reg_param.Ti
  Mux : Mux  Inputs=2
  Out1 : Outport
  wires:
  Constant1/1 -> Mux/2
  Mux/1 -> Out1/1
  Constant/1 -> Mux/1

== system Full_avg_converter/CV/DCM_CV_konstante ==
  Constant : Constant  Value=dcm_reg_param.KR
  Constant1 : Constant  Value=dcm_reg_param.KR/dcm_reg_param.Ti
  Mux : Mux  Inputs=2
  Out1 : Outport
  wires:
  Constant1/1 -> Mux/2
  Mux/1 -> Out1/1
  Constant/1 -> Mux/1

== system Full_avg_converter/CV/Generator signala poluvodičke sklopke ==
  IL : Inport
  Ir : Inport  Port=2
  Bistabil : spsBistableLib/Bistable  Qpriority=Set  ic=0  Ts=0
      settings: LibrarySourceBlock=sps_lib/Control/Bistable
  Constant1 : Constant  Value=sim_op.m0
  Komparator : RelationalOperator  Operator=<=  OutDataTypeStr=boolean  RndMeth=Simplest  InputSameDT=off
  Rampa : Integrator  ExternalReset=rising
  Subsystem : Subsystem  Commented=on
  Sum : Sum  Inputs=-+|
  T : DiscretePulseGenerator  PulseType=Time based  Period=boost.T
  upravljački sginal : Outport
  !Q : Outport  Port=2
  wires:
  Komparator/1 -> Bistabil/2
  Bistabil/2 -> !Q/1
  Bistabil/1 -> upravljački sginal/1
  IL/1 -> Komparator/2
  Sum/1 -> Komparator/1
  Ir/1 -> Sum/2
  Rampa/1 -> Sum/1
  T/1 -> Bistabil/1, Rampa/2
  Constant1/1 -> Rampa/1

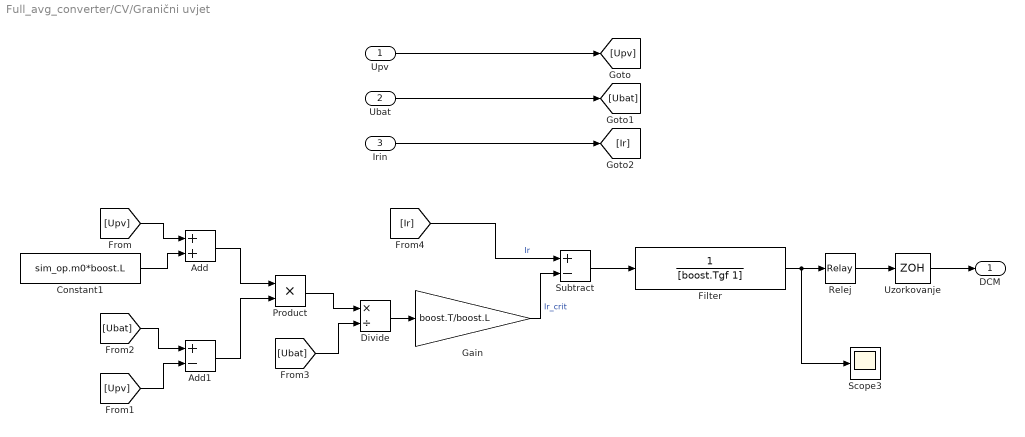
== system Full_avg_converter/CV/Granični uvjet ==
  Upv : Inport
  Ubat : Inport  Port=2
  Irin : Inport  Port=3
  Add : Sum
  Add1 : Sum  Inputs=+-
  Constant1 : Constant  Value=sim_op.m0*boost.L
  Divide : Product  Inputs=*/
  Filter : TransferFcn  Numerator=1  Denominator=[boost.Tgf 1]
  Gain : Gain  Gain=boost.T/boost.L
  Product : Product
  Relej : Relay  OnSwitchValue=0.01  OffSwitchValue=-0.01  OnOutputValue=0  OffOutputValue=1
  Scope3 : Scope
  Subtract : Sum  Inputs=+-
  Uzorkovanje : ZeroOrderHold  SampleTime=0.001
  DCM : Outport
  wires:
  Product/1 -> Divide/1
  Constant1/1 -> Add/2
  Add/1 -> Product/1
  Add1/1 -> Product/2
  Divide/1 -> Gain/1
  [Upv] -> Add/1
  [Upv] -> Add1/2
  [Ubat] -> Add1/1
  [Ubat] -> Divide/2
  Gain/1 -> Subtract/2  "Ir_crit"
  [Ir] -> Subtract/1  "Ir"
  Relej/1 -> Uzorkovanje/1
  Upv/1 -> [Upv]
  Ubat/1 -> [Ubat]
  Irin/1 -> [Ir]
  Subtract/1 -> Filter/1
  Filter/1 -> Scope3/1, Relej/1
  Uzorkovanje/1 -> DCM/1

== system Full_avg_converter/MPP/CCM_MPP_konstante ==
  Constant : Constant  Value=ccm_mpp_reg_param.KR
  Constant1 : Constant  Value=ccm_mpp_reg_param.KR/ccm_mpp_reg_param.Ti
  Mux : Mux  Inputs=2
  Out1 : Outport
  wires:
  Constant1/1 -> Mux/2
  Mux/1 -> Out1/1
  Constant/1 -> Mux/1

== system Full_avg_converter/MPP/DCM_MPP_konstante ==
  Constant : Constant  Value=dcm_mpp_reg_param.KR
  Constant1 : Constant  Value=dcm_mpp_reg_param.KR/dcm_mpp_reg_param.Ti
  Mux : Mux  Inputs=2
  Out1 : Outport
  wires:
  Constant1/1 -> Mux/2
  Mux/1 -> Out1/1
  Constant/1 -> Mux/1

== system Full_avg_converter/MPP/Generator signala poluvodičke sklopke ==
  IL : Inport
  Ir : Inport  Port=2
  Bistabil : spsBistableLib/Bistable  Qpriority=Set  ic=0  Ts=0
      settings: LibrarySourceBlock=sps_lib/Control/Bistable
  Constant1 : Constant  Value=sim_op.m0
  Komparator : RelationalOperator  Operator=<=  OutDataTypeStr=boolean  RndMeth=Simplest  InputSameDT=off
  Rampa : Integrator  ExternalReset=rising
  Subsystem : Subsystem  Commented=on
  Sum : Sum  Inputs=-+|
  T : DiscretePulseGenerator  PulseType=Time based  Period=boost.T
  upravljački sginal : Outport
  !Q : Outport  Port=2
  wires:
  Komparator/1 -> Bistabil/2
  Bistabil/2 -> !Q/1
  Bistabil/1 -> upravljački sginal/1
  IL/1 -> Komparator/2
  Sum/1 -> Komparator/1
  Ir/1 -> Sum/2
  Rampa/1 -> Sum/1
  T/1 -> Bistabil/1, Rampa/2
  Constant1/1 -> Rampa/1

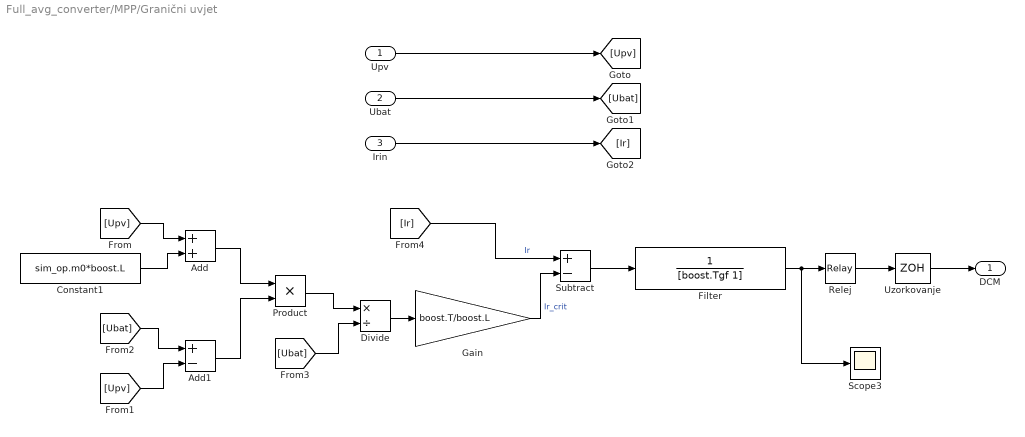
== system Full_avg_converter/MPP/Granični uvjet ==
  Upv : Inport
  Ubat : Inport  Port=2
  Irin : Inport  Port=3
  Add : Sum
  Add1 : Sum  Inputs=+-
  Constant1 : Constant  Value=sim_op.m0*boost.L
  Divide : Product  Inputs=*/
  Filter : TransferFcn  Numerator=1  Denominator=[boost.Tgf 1]
  Gain : Gain  Gain=boost.T/boost.L
  Product : Product
  Relej : Relay  OnSwitchValue=0.01  OffSwitchValue=-0.01  OnOutputValue=0  OffOutputValue=1
  Scope3 : Scope
  Subtract : Sum  Inputs=+-
  Uzorkovanje : ZeroOrderHold  SampleTime=0.001
  DCM : Outport
  wires:
  Product/1 -> Divide/1
  Constant1/1 -> Add/2
  Add/1 -> Product/1
  Add1/1 -> Product/2
  Divide/1 -> Gain/1
  [Upv] -> Add/1
  [Upv] -> Add1/2
  [Ubat] -> Add1/1
  [Ubat] -> Divide/2
  Gain/1 -> Subtract/2  "Ir_crit"
  [Ir] -> Subtract/1  "Ir"
  Relej/1 -> Uzorkovanje/1
  Upv/1 -> [Upv]
  Ubat/1 -> [Ubat]
  Irin/1 -> [Ir]
  Subtract/1 -> Filter/1
  Filter/1 -> Scope3/1, Relej/1
  Uzorkovanje/1 -> DCM/1

== system Full_avg_converter/Pretvarac/MOD_rada ==
  D : Inport
  Ubat : Inport  Port=2
  Upv : Inport  Port=3
  Clock : Clock
  Constant : Constant  Value=2
  Logical Operator : Logic  AllPortsSameDT=off  OutDataTypeStr=boolean
  Product : Product
  Relational Operator : RelationalOperator  Operator=<=  OutDataTypeStr=boolean  RndMeth=Simplest  InputSameDT=off
  Relational Operator1 : RelationalOperator  OutDataTypeStr=boolean  RndMeth=Simplest  InputSameDT=off
  Scope : Scope  NumInputPorts=2
  Subtract : Sum  Inputs=+-
  DISK : Outport  SampleTime=0.01
  wires:
  Ubat/1 -> Product/2, Subtract/1
  Upv/1 -> Subtract/2
  Relational Operator1/1 -> Logical Operator/1  "10s da se sustav ustali"
  Relational Operator/1 -> Logical Operator/2  "Uvjet za prelaz i diskontinuirani"
  Subtract/1 -> Scope/2, Relational Operator/2
  Product/1 -> Scope/1, Relational Operator/1
  Logical Operator/1 -> DISK/1
  Clock/1 -> Relational Operator1/1
  Constant/1 -> Relational Operator1/2
  D/1 -> Product/1

== system Full_avg_converter/Regulator/CV_konstante ==
  DCM : Inport
  CCM_param : Mux  Inputs=2
  Constant : Constant  Value=dcm_reg_param.KR
  Constant1 : Constant  Value=dcm_reg_param.KR/dcm_reg_param.Ti
  Constant2 : Constant  Value=ccm_reg_param.KR
  Constant3 : Constant  Value=ccm_reg_param.KR/ccm_reg_param.Ti
  DCM_param : Mux  Inputs=2
  Demux : Demux  Outputs=2
  Switch : Switch  Criteria=u2 > Threshold  SaturateOnIntegerOverflow=off  InputSameDT=off
  KR : Outport
  KR/Ti : Outport  Port=2
  wires:
  Constant/1 -> DCM_param/1
  Constant1/1 -> DCM_param/2
  DCM_param/1 -> Switch/1
  Constant2/1 -> CCM_param/1
  Constant3/1 -> CCM_param/2
  CCM_param/1 -> Switch/3
  DCM/1 -> Switch/2
  Switch/1 -> Demux/1
  Demux/1 -> KR/1
  Demux/2 -> KR/Ti/1

== system Full_avg_converter/Regulator/CV_limit ==
  Uoc : Inport
  Constant1 : Constant  Value=12
  Relational Operator : RelationalOperator  OutDataTypeStr=boolean  RndMeth=Simplest  InputSameDT=off
  CV_limit : Outport
  wires:
  Uoc/1 -> Relational Operator/1
  Constant1/1 -> Relational Operator/2
  Relational Operator/1 -> CV_limit/1

== system Full_avg_converter/Regulator/Generator signala poluvodičke sklopke ==
  IL : Inport
  Ir : Inport  Port=2
  Bistabil : spsBistableLib/Bistable  Qpriority=Set  ic=0  Ts=0
      settings: LibrarySourceBlock=sps_lib/Control/Bistable
  Constant1 : Constant  Value=sim_op.m0
  Komparator : RelationalOperator  Operator=<=  OutDataTypeStr=boolean  RndMeth=Simplest  InputSameDT=off
  Rampa : Integrator  ExternalReset=rising
  Subsystem : Subsystem  Commented=on
  Sum : Sum  Inputs=-+|
  T : DiscretePulseGenerator  PulseType=Time based  Period=boost.T
  upravljački sginal : Outport
  !Q : Outport  Port=2
  wires:
  Komparator/1 -> Bistabil/2
  Bistabil/2 -> !Q/1
  Bistabil/1 -> upravljački sginal/1
  IL/1 -> Komparator/2
  Sum/1 -> Komparator/1
  Ir/1 -> Sum/2
  Rampa/1 -> Sum/1
  T/1 -> Bistabil/1, Rampa/2
  Constant1/1 -> Rampa/1

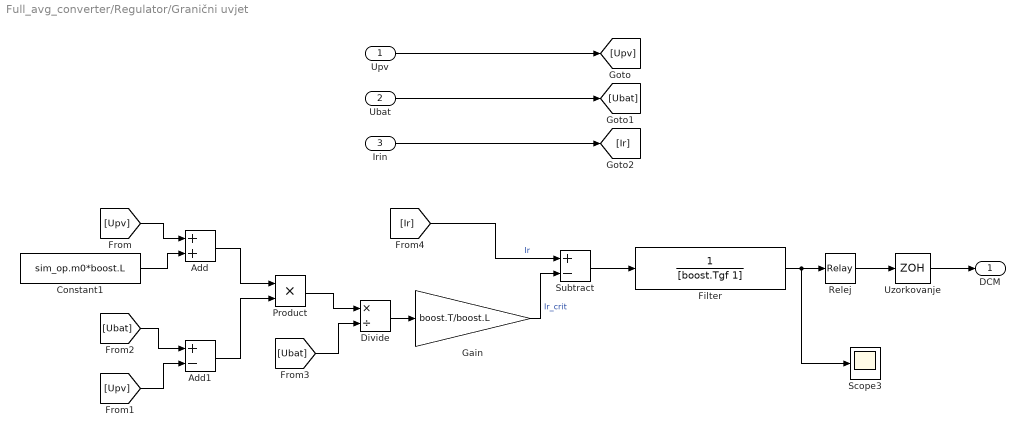
== system Full_avg_converter/Regulator/Granični uvjet ==
  Upv : Inport
  Ubat : Inport  Port=2
  Irin : Inport  Port=3
  Add : Sum
  Add1 : Sum  Inputs=+-
  Constant1 : Constant  Value=sim_op.m0*boost.L
  Divide : Product  Inputs=*/
  Filter : TransferFcn  Numerator=1  Denominator=[boost.Tgf 1]
  Gain : Gain  Gain=boost.T/boost.L
  Product : Product
  Relej : Relay  OnSwitchValue=0.01  OffSwitchValue=-0.01  OnOutputValue=0  OffOutputValue=1
  Scope3 : Scope
  Subtract : Sum  Inputs=+-
  Uzorkovanje : ZeroOrderHold  SampleTime=0.001
  DCM : Outport
  wires:
  Product/1 -> Divide/1
  Constant1/1 -> Add/2
  Add/1 -> Product/1
  Add1/1 -> Product/2
  Divide/1 -> Gain/1
  [Upv] -> Add/1
  [Upv] -> Add1/2
  [Ubat] -> Add1/1
  [Ubat] -> Divide/2
  Gain/1 -> Subtract/2  "Ir_crit"
  [Ir] -> Subtract/1  "Ir"
  Relej/1 -> Uzorkovanje/1
  Upv/1 -> [Upv]
  Ubat/1 -> [Ubat]
  Irin/1 -> [Ir]
  Subtract/1 -> Filter/1
  Filter/1 -> Scope3/1, Relej/1
  Uzorkovanje/1 -> DCM/1

== system Full_avg_converter/Regulator/MPP_konstante ==
  DCM : Inport
  CCM_param : Mux  Inputs=2
  Constant : Constant  Value=dcm_mpp_reg_param.KR
  Constant1 : Constant  Value=dcm_mpp_reg_param.KR/dcm_mpp_reg_param.Ti
  Constant2 : Constant  Value=ccm_mpp_reg_param.KR
  Constant3 : Constant  Value=ccm_mpp_reg_param.KR/ccm_mpp_reg_param.Ti
  DCM_param : Mux  Inputs=2
  Demux : Demux  Outputs=2
  Switch : Switch  Criteria=u2 > Threshold  SaturateOnIntegerOverflow=off  InputSameDT=off
  KR : Outport
  KR/Ti : Outport  Port=2
  wires:
  DCM_param/1 -> Switch/1
  CCM_param/1 -> Switch/3
  DCM/1 -> Switch/2
  Constant/1 -> DCM_param/1
  Constant1/1 -> DCM_param/2
  Constant2/1 -> CCM_param/1
  Constant3/1 -> CCM_param/2
  Switch/1 -> Demux/1
  Demux/1 -> KR/1
  Demux/2 -> KR/Ti/1

== system Full_avg_converter/Regulator/Subsystem ==
  Ir : Inport
  Upv : Inport  Port=2
  Ubat : Inport  Port=3
  CCM_D : Subsystem
  DCM_D : Subsystem
  Switch2 : Switch  Criteria=u2 > Threshold  SaturateOnIntegerOverflow=off  InputSameDT=off
  D : Outport
  wires:
  DCM_D/1(D) -> Switch2/1
  CCM_D/1(D) -> Switch2/3
  Switch2/1 -> D/1
  [DCM] -> Switch2/2
  Ubat/1 -> CCM_D/3(Ubat)
  Upv/1 -> CCM_D/2(Upv), DCM_D/2(Upv)
  Ir/1 -> CCM_D/1(Ir), DCM_D/1(Ir)

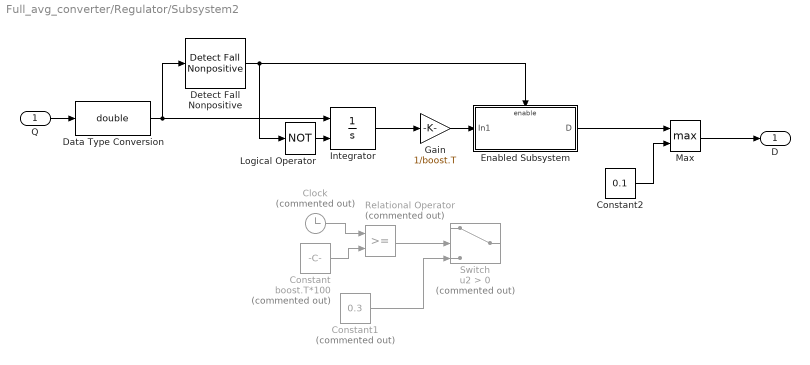
== system Full_avg_converter/Regulator/Subsystem2 ==
  Q : Inport
  Clock : Clock  Commented=on
  Constant : Constant  Commented=on  Value=boost.T*100
  Constant1 : Constant  Commented=on  Value=0.3
  Constant2 : Constant  Value=0.1
  Data Type Conversion : DataTypeConversion  OutDataTypeStr=double  SaturateOnIntegerOverflow=off  RndMeth=Floor
  Detect Fall Nonpositive : simulink/Logic and Bit Operations/Detect Fall Nonpositive  vinit=0  OutDataTypeStr=boolean
  Enabled Subsystem : Subsystem  TreatAsAtomicUnit=on
  Gain : Gain  Gain=1/boost.T
  Integrator : Integrator  ExternalReset=rising
  Logical Operator : Logic  Operator=NOT  AllPortsSameDT=off  OutDataTypeStr=boolean
  Max : MinMax  Function=max  Inputs=2
  Relational Operator : RelationalOperator  Commented=on  OutDataTypeStr=boolean  RndMeth=Simplest  InputSameDT=off
  Switch : Switch  Commented=on  Criteria=u2 > Threshold  SaturateOnIntegerOverflow=off  InputSameDT=off
  D : Outport
  wires:
  Integrator/1 -> Gain/1
  Gain/1 -> Enabled Subsystem/1(In1)
  Clock/1 -> Relational Operator/1
  Constant/1 -> Relational Operator/2
  Relational Operator/1 -> Switch/2
  Constant1/1 -> Switch/3
  Q/1 -> Data Type Conversion/1
  Data Type Conversion/1 -> Detect Fall Nonpositive/1, Integrator/1
  Logical Operator/1 -> Integrator/2
  Detect Fall Nonpositive/1 -> Logical Operator/1, Enabled Subsystem/Enable
  Enabled Subsystem/1(D) -> Max/1
  Max/1 -> D/1
  Constant2/1 -> Max/2

== system Full_avg_converter/CV/Generator signala poluvodičke sklopke/Subsystem ==
  Reset : Inport
  Ir_in : Inport  Port=2
  Add : Sum
  Compensation ramp switch : Switch  Criteria=u2 > Threshold  SaturateOnIntegerOverflow=off  InputSameDT=off
  Constant5 : Constant  Value=m0_ccm
  Constant6 : Constant  Value=Ramp
  Integrator : Integrator  ExternalReset=rising
  Scope : Scope
  Ir_out : Outport
  wires:
  Constant5/1 -> Integrator/1
  Integrator/1 -> Add/1
  Add/1 -> Compensation ramp switch/1
  Reset/1 -> Integrator/2
  Compensation ramp switch/1 -> Scope/1, Ir_out/1
  Constant6/1 -> Compensation ramp switch/2
  Ir_in/1 -> Compensation ramp switch/3, Add/2

== system Full_avg_converter/MPP/Generator signala poluvodičke sklopke/Subsystem ==
  Reset : Inport
  Ir_in : Inport  Port=2
  Add : Sum
  Compensation ramp switch : Switch  Criteria=u2 > Threshold  SaturateOnIntegerOverflow=off  InputSameDT=off
  Constant5 : Constant  Value=m0_ccm
  Constant6 : Constant  Value=Ramp
  Integrator : Integrator  ExternalReset=rising
  Scope : Scope
  Ir_out : Outport
  wires:
  Constant5/1 -> Integrator/1
  Integrator/1 -> Add/1
  Add/1 -> Compensation ramp switch/1
  Reset/1 -> Integrator/2
  Compensation ramp switch/1 -> Scope/1, Ir_out/1
  Constant6/1 -> Compensation ramp switch/2
  Ir_in/1 -> Compensation ramp switch/3, Add/2

== system Full_avg_converter/Regulator/Generator signala poluvodičke sklopke/Subsystem ==
  Reset : Inport
  Ir_in : Inport  Port=2
  Add : Sum
  Compensation ramp switch : Switch  Criteria=u2 > Threshold  SaturateOnIntegerOverflow=off  InputSameDT=off
  Constant5 : Constant  Value=m0_ccm
  Constant6 : Constant  Value=Ramp
  Integrator : Integrator  ExternalReset=rising
  Scope : Scope
  Ir_out : Outport
  wires:
  Constant5/1 -> Integrator/1
  Integrator/1 -> Add/1
  Add/1 -> Compensation ramp switch/1
  Reset/1 -> Integrator/2
  Compensation ramp switch/1 -> Scope/1, Ir_out/1
  Constant6/1 -> Compensation ramp switch/2
  Ir_in/1 -> Compensation ramp switch/3, Add/2

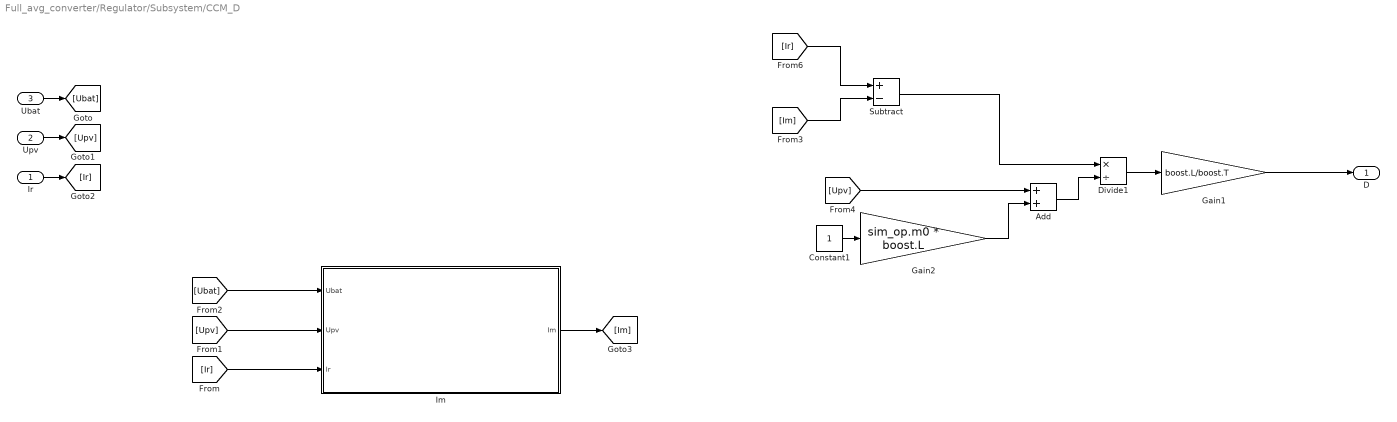
== system Full_avg_converter/Regulator/Subsystem/CCM_D ==
  Ir : Inport
  Upv : Inport  Port=2
  Ubat : Inport  Port=3
  Add : Sum
  Constant1 : Constant
  Divide1 : Product  Inputs=*/
  Gain1 : Gain  Gain=boost.L/boost.T
  Gain2 : Gain  Gain=sim_op.m0 * boost.L
  Im : Subsystem
  Subtract : Sum  Inputs=+-
  D : Outport
  wires:
  Ubat/1 -> [Ubat]
  Upv/1 -> [Upv]
  Ir/1 -> [Ir]
  [Ubat] -> Im/1(Ubat)
  [Upv] -> Im/2(Upv)
  [Ir] -> Im/3(Ir)
  Im/1(Im) -> [Im]
  Gain2/1 -> Add/2
  Gain1/1 -> D/1
  [Upv] -> Add/1
  Divide1/1 -> Gain1/1
  Constant1/1 -> Gain2/1
  Add/1 -> Divide1/2
  Subtract/1 -> Divide1/1
  [Ir] -> Subtract/1
  [Im] -> Subtract/2

== system Full_avg_converter/Regulator/Subsystem/DCM_D ==
  Ir : Inport
  Upv : Inport  Port=2
  Add : Sum
  Constant1 : Constant
  Divide : Product  Inputs=*/
  Gain : Gain  Gain=boost.L/boost.T
  Gain1 : Gain  Gain=sim_op.m0 * boost.L
  D : Outport
  wires:
  Constant1/1 -> Gain1/1
  Gain1/1 -> Add/2
  Add/1 -> Divide/2
  Divide/1 -> Gain/1
  Gain/1 -> D/1
  Upv/1 -> Add/1
  Ir/1 -> Divide/1

== system Full_avg_converter/Regulator/Subsystem2/Enabled Subsystem ==
  In1 : Inport
  Enable : EnablePort
  D : Outport
  wires:
  In1/1 -> D/1

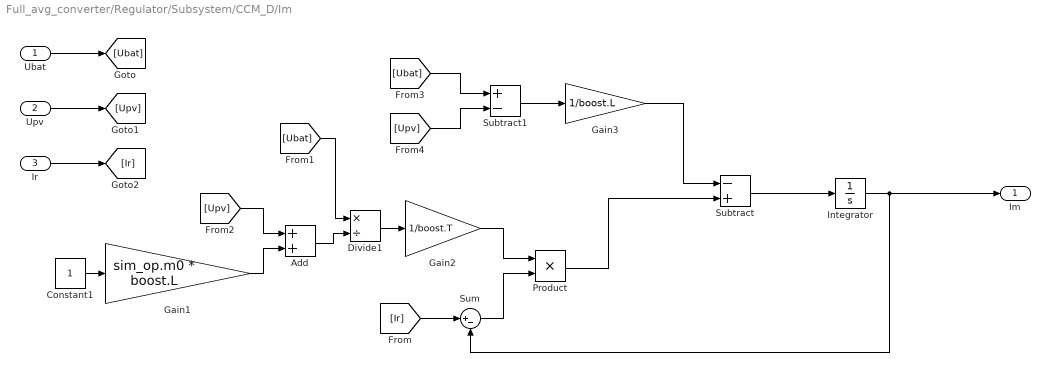
== system Full_avg_converter/Regulator/Subsystem/CCM_D/Im ==
  Ubat : Inport
  Upv : Inport  Port=2
  Ir : Inport  Port=3
  Add : Sum
  Constant1 : Constant
  Divide1 : Product  Inputs=*/
  Gain1 : Gain  Gain=sim_op.m0 * boost.L
  Gain2 : Gain  Gain=1/boost.T
  Gain3 : Gain  Gain=1/boost.L
  Integrator : Integrator
  Product : Product
  Subtract : Sum  Inputs=-+
  Subtract1 : Sum  Inputs=+-
  Sum : Sum  Inputs=|+-
  Im : Outport
  wires:
  Sum/1 -> Product/2
  Divide1/1 -> Gain2/1
  Product/1 -> Subtract/2
  Add/1 -> Divide1/2
  Subtract/1 -> Integrator/1
  [Ubat] -> Subtract1/1
  Subtract1/1 -> Gain3/1
  [Upv] -> Subtract1/2
  Gain2/1 -> Product/1
  Integrator/1 -> Im/1, Sum/2
  Constant1/1 -> Gain1/1
  Gain1/1 -> Add/2
  [Ir] -> Sum/1
  Gain3/1 -> Subtract/1
  Ubat/1 -> [Ubat]
  Upv/1 -> [Upv]
  Ir/1 -> [Ir]
  [Upv] -> Add/1
  [Ubat] -> Divide1/1

== matlab function Full_avg_converter/Regulator/MATLAB Function ==
  data: Upv1 input; Upvref output; Upv2 input; Ipv1 input; Ipv2 input
function Upvref = mppt_my3(Upv1, Upv2, Ipv1, Ipv2)
% MPPT incremental conductance (hybrid) with robust numerics and anti-stall
% Inputs:  Upv1, Upv2  - PV voltage samples (previous, current) [V]
%          Ipv1, Ipv2  - PV current samples (previous, current) [A]
% Outputs: Upvref      - next PV voltage reference [V]
%          step        - applied step (Upvref - Upv2) [V]

% ---- Tunables ----
dU_small     = 0.01;     % [V] threshold for safe derivative fallback
zero_thresh  = 1e-4;     % [V]/[A] "no change" threshold
epsilon      = 1e-3;     % [W/V] near-zero slope threshold
k_step       = 20;       % step gain: V per (W/V)
step_min     = 0.01;     % [V] minimum perturb to avoid stalling
step_max     = 0.2;      % [V] maximum step magnitude
Umin         = 4.0;      % [V] lower clamp
Umax         = 6.2;      % [V] upper clamp
I_dark       = 1e-3;     % [A] "no irradiance" threshold

% Default: start from current voltage
Upvref = Upv2;

% ---- Safety clamps on input reference base ----
if Upvref < Umin
    Upvref = Umin;
elseif Upvref > Umax
    Upvref = Umax;
end

% ---- Dark / near-zero current handling ----
% If essentially no PV current, gently reduce reference to seek a valid point
if (Ipv1 <= I_dark) && (Ipv2 <= I_dark)
    Upvref = max(Umin, 0.9 * Upv2);
    return;
end

% ---- Differences ----
dUpv = Upv1 - Upv2;
dIpv = Ipv1 - Ipv2;

% If both changes are tiny, do a small dither (prevents freezing on noise)
if (abs(dUpv) < zero_thresh) && (abs(dIpv) < zero_thresh)
    Upvref = clamp(Upv2 + step_min, Umin, Umax);
    return;
end

% ---- Compute dP/dU robustly ----
% dP/dU = I + U * dI/dU
if abs(dUpv) > dU_small
    dIdU = dIpv / dUpv;
    dPdU = Ipv1 + Upv1 * dIdU;
else
    % Fallback: approximate slope by delta power / delta voltage direction
    % If voltage barely changed, use delta current sign as proxy
    dPdU = (Ipv1 - Ipv2);
end

% ---- Decide step ----
if abs(dPdU) > epsilon
    step_var = min(step_max, k_step * abs(dPdU));
    Upvref   = Upv2 + sign(dPdU) * step_var;
else
    % Near MPP: keep a tiny perturb so it doesn't stall
    % Use the last voltage direction if available; otherwise push up
    dir = 1;
    if abs(dUpv) > zero_thresh
        dir = sign(dUpv);
        if dir == 0, dir = 1; end
    end
    Upvref = Upv2 + dir * step_min;
end

% ---- Final clamp + output ----
Upvref = clamp(Upvref, Umin, Umax);

end

% Local helper (works in MATLAB R2016b+ as local function)
function y = clamp(x, lo, hi)
y = min(hi, max(lo, x));
end
